simulink model "ee145L3p1"  (R2019a)
settings: Solver=VariableStepAuto  StartTime=0.0  StopTime=10.0  RelTol=1e-3
libraries: simulink x2
settings Model: OrderedModelArguments=off  Creator=sk  LastModifiedBy=sk

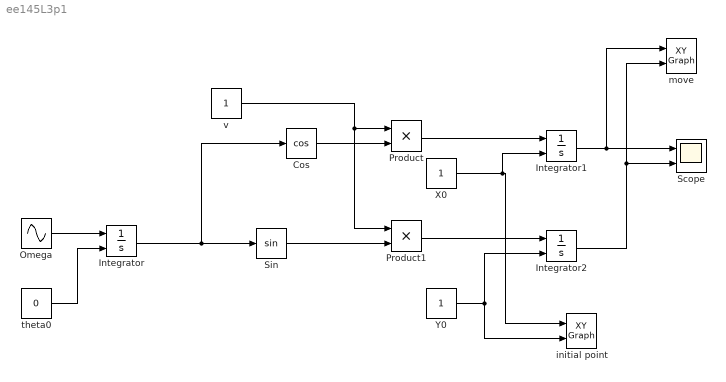
== system ee145L3p1 ==
  Cos : Trigonometry  Operator=cos
  Integrator : Integrator  InitialConditionSource=external
  Integrator1 : Integrator  InitialConditionSource=external
  Integrator2 : Integrator  InitialConditionSource=external
  Omega : Sin  Frequency=.01  SampleTime=0
  Product : Product
  Product1 : Product
  Scope : Scope  NumInputPorts=2
  Sin : Trigonometry
  "X0 " : Constant
  Y0 : Constant
  "initial point " : simulink/Sinks/XY Graph  xmin=0  xmax=5  ymin=0  ymax=5  st=-1
  move : simulink/Sinks/XY Graph  xmin=0  xmax=5  ymin=0  ymax=5  st=-1
  "theta0 " : Constant  Value=0
  "v " : Constant
  wires:
  "v "/1 -> Product1/1, Product/1
  Integrator/1 -> Cos/1, Sin/1
  Omega/1 -> Integrator/1
  "theta0 "/1 -> Integrator/2
  "X0 "/1 -> "initial point "/1, Integrator1/2
  Y0/1 -> "initial point "/2, Integrator2/2
  Integrator1/1 -> move/1, Scope/1
  Product/1 -> Integrator1/1
  Integrator2/1 -> move/2, Scope/2
  Cos/1 -> Product/2
  Product1/1 -> Integrator2/1
  Sin/1 -> Product1/2
